simulink model "sun"  (R2023a)
settings: Solver=ode4  StartTime=0.0  StopTime=10.0  FixedStep=dt  RelTol=1e-3
settings Model: Creator=ndelurgio  LastModifiedBy=ndelurgio

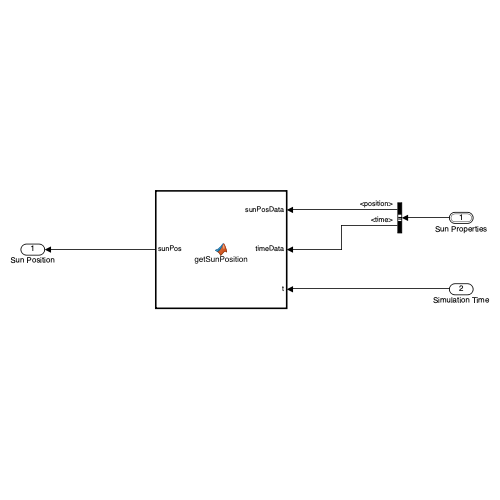
[thumbnail: Simulink's stored preview of the top-level diagram]
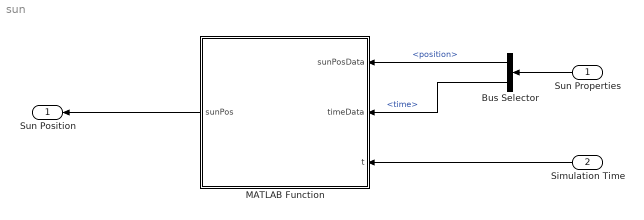
== system sun ==
  Sun Properties : Inport  OutDataTypeStr=Bus: sunProperties
  Simulation Time : Inport  Port=2
  Bus Selector : BusSelector  OutputSignals=position,time
  MATLAB Function : MATLAB Function  TreatAsAtomicUnit=on
  Sun Position : Outport
  wires:
  Sun Properties/1 -> Bus Selector/1
  Bus Selector/1 -> MATLAB Function/1(sunPosData)  "<position>"
  Bus Selector/2 -> MATLAB Function/2(timeData)  "<time>"
  Simulation Time/1 -> MATLAB Function/3(t)
  MATLAB Function/1(sunPos) -> Sun Position/1

== matlab function sun/MATLAB Function ==
  data: sunPosData input; sunPos output; timeData input; t input
function sunPos = getSunPosition(sunPosData,timeData,t)

sunPos = getSunPosition(sunPosData,timeData,t);

end
